simulink library "ADCS_lib"  (R2019a)
settings: Solver=VariableStepAuto  StartTime=0.0  StopTime=10.0  RelTol=1e-3
undefined symbols (not defined in the file): D_distri, G_g, G_s, G_t, Gs, I_rw, I_vscmg, I_w, J_w, K, Kc, Ki, Kp, Kv, m, OMEGA_0, P, quat_0, smiData, X, Y, Z
libraries: sm_lib x31, aerolibutil x15, nesl_utility x13, sharedtransform x4, $bdroot x2
(part 3 of 3)

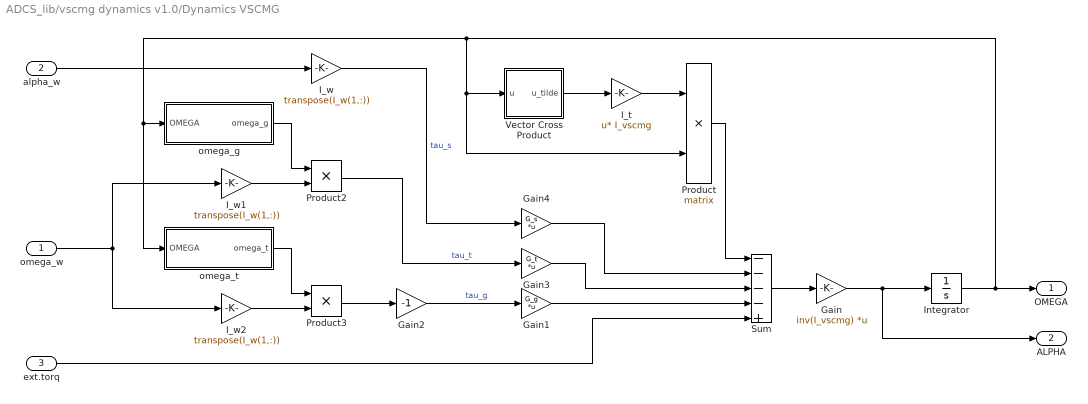
== system ADCS_lib/vscmg dynamics v1.0/Dynamics VSCMG ==
  omega_w : Inport
  alpha_w : Inport  Port=2
  ext.torq : Inport  Port=3
  Gain : Gain  Gain=inv(I_vscmg)  Multiplication=Matrix(K*u)
  Gain1 : Gain  Gain=G_g  Multiplication=Matrix(K*u)
  Gain2 : Gain  Gain=-1
  Gain3 : Gain  Gain=G_t  Multiplication=Matrix(K*u)
  Gain4 : Gain  Gain=G_s  Multiplication=Matrix(K*u)
  I_t : Gain  Gain=I_vscmg  Multiplication=Matrix(u*K)
  I_w : Gain  Gain=transpose(I_w(1,:))
  I_w1 : Gain  Gain=transpose(I_w(1,:))
  I_w2 : Gain  Gain=transpose(I_w(1,:))
  Integrator : Integrator  InitialCondition=OMEGA_0
  Product : Product  Multiplication=Matrix(*)
  Product2 : Product
  Product3 : Product
  Sum : Sum  Inputs=----+
  Vector Cross Product : MATLAB Function  TreatAsAtomicUnit=on
  omega_g : Subsystem
  omega_t : Subsystem
  OMEGA : Outport
  ALPHA : Outport  Port=2
  wires:
  Sum/1 -> Gain/1
  Gain/1 -> Integrator/1, ALPHA/1
  Integrator/1 -> omega_g/1(OMEGA), omega_t/1(OMEGA), Product/2, Vector Cross Product/1(u), OMEGA/1
  Vector Cross Product/1(u_tilde) -> I_t/1
  I_t/1 -> Product/1
  Product/1 -> Sum/1
  ext.torq/1 -> Sum/5
  alpha_w/1 -> I_w/1
  I_w/1 -> Gain4/1  "tau_s"
  I_w1/1 -> Product2/2
  omega_g/1(omega_g) -> Product2/1
  omega_t/1(omega_t) -> Product3/1
  I_w2/1 -> Product3/2
  omega_w/1 -> I_w1/1, I_w2/1
  Product3/1 -> Gain2/1
  Gain2/1 -> Gain1/1  "tau_g"
  Product2/1 -> Gain3/1  "tau_t"
  Gain1/1 -> Sum/4
  Gain3/1 -> Sum/3
  Gain4/1 -> Sum/2

== system ADCS_lib/vscmg dynamics v1.0/Kinematics1 ==
  OMEGA : Inport
  Constant : Constant  Value=0
  Gain : Gain  Gain=0.5
  Integrator : Integrator  InitialCondition=quat_0
  Quaternion Multiplication : aerolibutil/Quaternion Multiplication
  Vector Concatenate : Concatenate
  q : Outport
  wires:
  Constant/1 -> Vector Concatenate/1
  Vector Concatenate/1 -> Quaternion Multiplication/2
  Gain/1 -> Quaternion Multiplication/1
  Integrator/1 -> Gain/1, q/1
  OMEGA/1 -> Vector Concatenate/2
  Quaternion Multiplication/1 -> Integrator/1

== system ADCS_lib/vscmg dynamics v1.0/VSCMGC ==
  ALPHA : Inport
  tau_cmd : Inport  Port=2
  Demux : Demux
  Distri Mtx2 : Gain  Gain=D_distri  Multiplication=Matrix(K*u)
  Mux1 : Mux
  Mux2 : Mux
  RW 1 : Subsystem
  RW 2 : Subsystem
  RW 3 : Subsystem
  RW 4 : Subsystem
  omega_w : Outport
  alpha_w : Outport  Port=2
  wires:
  Demux/3 -> RW 3/2(u_s_3)
  Demux/1 -> RW 1/2(u_s_1)
  Demux/2 -> RW 2/2(u_s_2)
  Demux/4 -> RW 4/2(u_s_4)
  tau_cmd/1 -> Distri Mtx2/1
  ALPHA/1 -> RW 4/1(ALPHA), RW 3/1(ALPHA), RW 2/1(ALPHA), RW 1/1(ALPHA)
  Distri Mtx2/1 -> Demux/1  "u_s"
  Mux1/1 -> alpha_w/1
  Mux2/1 -> omega_w/1
  RW 1/1(omega_w_1) -> Mux2/1
  RW 2/1(omega_w_2) -> Mux2/2
  RW 3/1(omega_w_3) -> Mux2/3
  RW 4/1(omega_w_4) -> Mux2/4
  RW 1/2(alpha_w_1) -> Mux1/1
  RW 2/2(alpha_w_2) -> Mux1/2
  RW 3/2(alpha_w_3) -> Mux1/3
  RW 4/2(alpha_w_4) -> Mux1/4

== system ADCS_lib/Actuator/Reaction Wheel Cluster/RW 1 ==
  OMEGA : Inport
  ALPHA : Inport  Port=2
  u_s_1 : Inport  Port=3
  Gain : Gain  Gain=1/I_w(1,1)
  Gain1 : Gain  Gain=G_s(:,1).'  Multiplication=Matrix(K*u)
  Gain2 : Gain  Gain=G_s(:,1).'  Multiplication=Matrix(K*u)
  I_w : Gain  Gain=I_w(1,1)
  Integrator : Integrator
  Sum : Sum  Inputs=+-
  Sum1 : Sum
  h_w_1 : Outport
  omega_w_1 : Outport  Port=2
  wires:
  Sum/1 -> Integrator/1
  Integrator/1 -> Sum1/2, omega_w_1/1
  u_s_1/1 -> Gain/1
  Gain/1 -> Sum/1
  Gain1/1 -> Sum/2
  ALPHA/1 -> Gain1/1
  Sum1/1 -> I_w/1
  I_w/1 -> h_w_1/1
  Gain2/1 -> Sum1/1
  OMEGA/1 -> Gain2/1

== system ADCS_lib/Actuator/Reaction Wheel Cluster/RW 2 ==
  OMEGA : Inport
  ALPHA : Inport  Port=2
  u_s_2 : Inport  Port=3
  Gain : Gain  Gain=1/I_w(1,2)
  Gain1 : Gain  Gain=G_s(:,2).'  Multiplication=Matrix(K*u)
  Gain2 : Gain  Gain=G_s(:,2).'  Multiplication=Matrix(K*u)
  I_w : Gain  Gain=I_w(1,2)
  Integrator : Integrator
  Sum : Sum  Inputs=+-
  Sum1 : Sum
  h_w_2 : Outport
  omega_w_2 : Outport  Port=2
  wires:
  OMEGA/1 -> Gain2/1
  Gain2/1 -> Sum1/1
  I_w/1 -> h_w_2/1
  Sum1/1 -> I_w/1
  ALPHA/1 -> Gain1/1
  Gain1/1 -> Sum/2
  Gain/1 -> Sum/1
  u_s_2/1 -> Gain/1
  Integrator/1 -> omega_w_2/1, Sum1/2
  Sum/1 -> Integrator/1

== system ADCS_lib/Actuator/Reaction Wheel Cluster/RW 3 ==
  OMEGA : Inport
  ALPHA : Inport  Port=2
  u_s_3 : Inport  Port=3
  Gain : Gain  Gain=1/I_w(1,3)
  Gain1 : Gain  Gain=G_s(:,3).'  Multiplication=Matrix(K*u)
  Gain2 : Gain  Gain=G_s(:,3).'  Multiplication=Matrix(K*u)
  I_w : Gain  Gain=I_w(1,3)
  Integrator : Integrator
  Sum : Sum  Inputs=+-
  Sum1 : Sum
  h_w_3 : Outport
  omega_w_3 : Outport  Port=2
  wires:
  Sum/1 -> Integrator/1
  Integrator/1 -> Sum1/2, omega_w_3/1
  u_s_3/1 -> Gain/1
  Gain/1 -> Sum/1
  Gain1/1 -> Sum/2
  ALPHA/1 -> Gain1/1
  Sum1/1 -> I_w/1
  I_w/1 -> h_w_3/1
  Gain2/1 -> Sum1/1
  OMEGA/1 -> Gain2/1

== system ADCS_lib/Actuator/Reaction Wheel Cluster/RW 4 ==
  OMEGA : Inport
  ALPHA : Inport  Port=2
  u_s_4 : Inport  Port=3
  Gain : Gain  Gain=1/I_w(1,4)
  Gain1 : Gain  Gain=G_s(:,4).'  Multiplication=Matrix(K*u)
  Gain2 : Gain  Gain=G_s(:,4).'  Multiplication=Matrix(K*u)
  I_w : Gain  Gain=I_w(1,4)
  Integrator : Integrator
  Sum : Sum  Inputs=+-
  Sum1 : Sum
  h_w_4 : Outport
  omega_w_4 : Outport  Port=2
  wires:
  OMEGA/1 -> Gain2/1
  Gain2/1 -> Sum1/1
  I_w/1 -> h_w_4/1
  Sum1/1 -> I_w/1
  ALPHA/1 -> Gain1/1
  Gain1/1 -> Sum/2
  Gain/1 -> Sum/1
  u_s_4/1 -> Gain/1
  Integrator/1 -> omega_w_4/1, Sum1/2
  Sum/1 -> Integrator/1

== system ADCS_lib/LQI_Full State_Verified1/Vector Out Unwinding1/Short Rotation ==
  q : Inport
  Gain1 : Gain  Gain=-1
  Sign1 : Signum
  extract scalar part : Selector  InputPortWidth=4  IndexOptions=Index vector (dialog)  Indices=[1]  OutputSizes=1
  sgn : Outport
  wires:
  Gain1/1 -> sgn/1
  Sign1/1 -> Gain1/1
  extract scalar part/1 -> Sign1/1
  q/1 -> extract scalar part/1

== system ADCS_lib/LQI_Half State_Don't Use!/Vector Out Unwinding2/Short Rotation ==
  q : Inport
  Gain1 : Gain  Gain=-1
  Sign1 : Signum
  extract scalar part : Selector  InputPortWidth=4  IndexOptions=Index vector (dialog)  Indices=[1]  OutputSizes=1
  sgn : Outport
  wires:
  q/1 -> extract scalar part/1
  extract scalar part/1 -> Sign1/1
  Sign1/1 -> Gain1/1
  Gain1/1 -> sgn/1

== system ADCS_lib/LQR Compensated_Verified/Vector Out Unwinding/Short Rotation ==
  q : Inport
  Gain1 : Gain  Gain=-1
  Sign1 : Signum
  extract scalar part : Selector  InputPortWidth=4  IndexOptions=Index vector (dialog)  Indices=[1]  OutputSizes=1
  sgn : Outport
  wires:
  q/1 -> extract scalar part/1
  extract scalar part/1 -> Sign1/1
  Sign1/1 -> Gain1/1
  Gain1/1 -> sgn/1

== system ADCS_lib/PIV Compact_Verified/Vector Out Unwinding/Short Rotation ==
  q : Inport
  Gain1 : Gain  Gain=-1
  Sign1 : Signum
  extract scalar part : Selector  InputPortWidth=4  IndexOptions=Index vector (dialog)  Indices=[1]  OutputSizes=1
  sgn : Outport
  wires:
  q/1 -> extract scalar part/1
  extract scalar part/1 -> Sign1/1
  Sign1/1 -> Gain1/1
  Gain1/1 -> sgn/1

== system ADCS_lib/PIV Compact_Verified/Vector Out Unwinding1/Short Rotation ==
  q : Inport
  Gain1 : Gain  Gain=-1
  Sign1 : Signum
  extract scalar part : Selector  InputPortWidth=4  IndexOptions=Index vector (dialog)  Indices=[1]  OutputSizes=1
  sgn : Outport
  wires:
  Gain1/1 -> sgn/1
  Sign1/1 -> Gain1/1
  extract scalar part/1 -> Sign1/1
  q/1 -> extract scalar part/1

== system ADCS_lib/vscmg dynamics v1.0/Dynamics VSCMG/omega_g ==
  OMEGA : Inport
  Gain : Gain  Gain=transpose(G_g(:,1))  Multiplication=Matrix(K*u)
  Gain1 : Gain  Gain=transpose(G_g(:,2))  Multiplication=Matrix(K*u)
  Gain2 : Gain  Gain=transpose(G_g(:,3))  Multiplication=Matrix(K*u)
  Gain3 : Gain  Gain=transpose(G_g(:,4))  Multiplication=Matrix(K*u)
  Mux : Mux
  omega_g : Outport
  wires:
  Mux/1 -> omega_g/1
  Gain3/1 -> Mux/4
  Gain2/1 -> Mux/3
  Gain1/1 -> Mux/2
  Gain/1 -> Mux/1
  OMEGA/1 -> Gain/1, Gain1/1, Gain2/1, Gain3/1

== system ADCS_lib/vscmg dynamics v1.0/Dynamics VSCMG/omega_t ==
  OMEGA : Inport
  Gain : Gain  Gain=transpose(G_t(:,1))  Multiplication=Matrix(K*u)
  Gain1 : Gain  Gain=transpose(G_t(:,2))  Multiplication=Matrix(K*u)
  Gain2 : Gain  Gain=transpose(G_t(:,3))  Multiplication=Matrix(K*u)
  Gain3 : Gain  Gain=transpose(G_t(:,4))  Multiplication=Matrix(K*u)
  Mux : Mux
  omega_t : Outport
  wires:
  OMEGA/1 -> Gain3/1, Gain2/1, Gain1/1, Gain/1
  Gain/1 -> Mux/1
  Gain1/1 -> Mux/2
  Gain2/1 -> Mux/3
  Gain3/1 -> Mux/4
  Mux/1 -> omega_t/1

== system ADCS_lib/vscmg dynamics v1.0/VSCMGC/RW 1 ==
  ALPHA : Inport
  u_s_1 : Inport  Port=2
  Gain : Gain  Gain=1/I_w(1,1)
  Gain1 : Gain  Gain=G_s(:,1).'  Multiplication=Matrix(K*u)
  Integrator : Integrator
  Sum : Sum  Inputs=+-
  omega_w_1 : Outport
  alpha_w_1 : Outport  Port=2
  wires:
  Sum/1 -> alpha_w_1/1, Integrator/1
  Integrator/1 -> omega_w_1/1
  u_s_1/1 -> Gain/1
  Gain/1 -> Sum/1
  Gain1/1 -> Sum/2
  ALPHA/1 -> Gain1/1

== system ADCS_lib/vscmg dynamics v1.0/VSCMGC/RW 2 ==
  ALPHA : Inport
  u_s_2 : Inport  Port=2
  Gain : Gain  Gain=1/I_w(1,2)
  Gain1 : Gain  Gain=G_s(:,2).'  Multiplication=Matrix(K*u)
  Integrator : Integrator
  Sum : Sum  Inputs=+-
  omega_w_2 : Outport
  alpha_w_2 : Outport  Port=2
  wires:
  ALPHA/1 -> Gain1/1
  Gain1/1 -> Sum/2
  Gain/1 -> Sum/1
  u_s_2/1 -> Gain/1
  Integrator/1 -> omega_w_2/1
  Sum/1 -> alpha_w_2/1, Integrator/1

== system ADCS_lib/vscmg dynamics v1.0/VSCMGC/RW 3 ==
  ALPHA : Inport
  u_s_3 : Inport  Port=2
  Gain : Gain  Gain=1/I_w(1,3)
  Gain1 : Gain  Gain=G_s(:,3).'  Multiplication=Matrix(K*u)
  Integrator : Integrator
  Sum : Sum  Inputs=+-
  omega_w_3 : Outport
  alpha_w_3 : Outport  Port=2
  wires:
  Sum/1 -> alpha_w_3/1, Integrator/1
  Integrator/1 -> omega_w_3/1
  u_s_3/1 -> Gain/1
  Gain/1 -> Sum/1
  Gain1/1 -> Sum/2
  ALPHA/1 -> Gain1/1

== system ADCS_lib/vscmg dynamics v1.0/VSCMGC/RW 4 ==
  ALPHA : Inport
  u_s_4 : Inport  Port=2
  Gain : Gain  Gain=1/I_w(1,4)
  Gain1 : Gain  Gain=G_s(:,4).'  Multiplication=Matrix(K*u)
  Integrator : Integrator
  Sum : Sum  Inputs=+-
  omega_w_4 : Outport
  alpha_w_4 : Outport  Port=2
  wires:
  ALPHA/1 -> Gain1/1
  Gain1/1 -> Sum/2
  Gain/1 -> Sum/1
  u_s_4/1 -> Gain/1
  Integrator/1 -> omega_w_4/1
  Sum/1 -> alpha_w_4/1, Integrator/1

== matlab function ADCS_lib/Reaction Wheel ==
  data: ALPHA input; tau_wheel output; u_s_cmd input; index input; omega_wheel output; h_wheel output
function [tau_wheel,omega_wheel,h_wheel] = RW(ALPHA,u_s_cmd,index)

tau_wheel = u_s_cmd-J_w(1,index)*(transpose(Gs(:,index))*ALPHA);
omega_wheel = (tau_wheel^2)/(2*J_w(1,index));
h_wheel = J_w(1,index)*omega_wheel;

== matlab function ADCS_lib/QuEST ==
  data: V_N input; BN output size=[4 1]; V_B input; WT input
function BN = quest(V_N,V_B,WT)
B = zeros(3);

% count # of sensors
dim = size(V_N); 
n_sensor = dim(2);

% normalize V_N
for n = 1:n_sensor
    V_N(:,n)=V_N(:,n)/norm(V_N(:,n));
end
    
% normalize V_B
for n = 1:n_sensor
    V_B(:,n)=V_B(:,n)/norm(V_B(:,n));
end

% assemble K matrix
for n = 1:n_sensor
    B=WT(n)*V_B(:,n)*transpose(V_N(:,n))+B;
end
S = B+transpose(B);
sigma = trace(B);
Z = [B(2,3)-B(3,2);
     B(3,1)-B(1,3);
     B(1,2)-B(2,1)];
K = [sigma transpose(Z);Z S-sigma*eye(3)];

% optimize eigenvalue
lambda = sum(WT); % first guess
for i = 1:2
    f = det(K-lambda*eye(4));
    f_dash = det(K-lambda*eye(4))*trace(inv(K-lambda*eye(4))*-eye(4));
    lambda = lambda - (f/f_dash);
end

% compute Rodrigues parameter & convert to Quaternion
q = inv((lambda+sigma)*eye(3)-S)*Z;
quatr = [1;q]/sqrt(1+transpose(q)*q);

BN = quatr;

== matlab function ADCS_lib/Reaction Wheel Cluster/Reaction Wheel 1 ==
  data: ALPHA input; tau_wheel output; u_s_cmd input; index input; omega_wheel output; h_wheel output
function [tau_wheel,omega_wheel,h_wheel] = RW(ALPHA,u_s_cmd,index)

tau_wheel = u_s_cmd-J_w(1,index)*(transpose(Gs(:,index))*ALPHA);
omega_wheel = (tau_wheel^2)/(2*J_w(1,index));
h_wheel = J_w(1,index)*omega_wheel;

== matlab function ADCS_lib/Reaction Wheel Cluster/Reaction Wheel 2 ==
  data: ALPHA input; tau_wheel output; u_s_cmd input; index input; omega_wheel output; h_wheel output
function [tau_wheel,omega_wheel,h_wheel] = RW(ALPHA,u_s_cmd,index)

tau_wheel = u_s_cmd-J_w(1,index)*(transpose(Gs(:,index))*ALPHA);
omega_wheel = (tau_wheel^2)/(2*J_w(1,index));
h_wheel = J_w(1,index)*omega_wheel;

== matlab function ADCS_lib/Reaction Wheel Cluster/Reaction Wheel 3 ==
  data: ALPHA input; tau_wheel output; u_s_cmd input; index input; omega_wheel output; h_wheel output
function [tau_wheel,omega_wheel,h_wheel] = RW(ALPHA,u_s_cmd,index)

tau_wheel = u_s_cmd-J_w(1,index)*(transpose(Gs(:,index))*ALPHA);
omega_wheel = (tau_wheel^2)/(2*J_w(1,index));
h_wheel = J_w(1,index)*omega_wheel;

== matlab function ADCS_lib/Reaction Wheel Cluster/Reaction Wheel 4 ==
  data: ALPHA input; tau_wheel output; u_s_cmd input; index input; omega_wheel output; h_wheel output
function [tau_wheel,omega_wheel,h_wheel] = RW(ALPHA,u_s_cmd,index)

tau_wheel = u_s_cmd-J_w(1,index)*(transpose(Gs(:,index))*ALPHA);
omega_wheel = (tau_wheel^2)/(2*J_w(1,index));
h_wheel = J_w(1,index)*omega_wheel;

== matlab function ADCS_lib/tilde_cross P ==
  data: u input; u_tilde output
function u_tilde = tilde(u)
u_tilde = [0 -u(3) u(2);
           u(3) 0 -u(1);
           -u(2) u(1) 0];

== matlab function ADCS_lib/Satellite Dynamics/Equation of Motion ==
  data: OMEGA input; ALPHA output; h_app_RWC input; tau_app_RWC input; tau_app_distrb input
function ALPHA = dynamics(OMEGA,h_app_RWC,tau_app_RWC,tau_app_distrb)

% assemble OMEGA_tilde for cross product
OMEGA_tilde = [0 -OMEGA(3) OMEGA(2);
               OMEGA(3) 0 -OMEGA(1);
              -OMEGA(2) OMEGA(1) 0];
          
% calculate ALPHA
ALPHA = inv(I_tot) * (-OMEGA_tilde*I_tot*OMEGA - tau_app_RWC - OMEGA_tilde*h_app_RWC + tau_app_distrb)

== matlab function ADCS_lib/Dynamics1/Vector Cross Product ==
  data: u input; u_tilde output
function u_tilde = tilde(u)
u_tilde = [0 -u(3) u(2);
           u(3) 0 -u(1);
           -u(2) u(1) 0];

== matlab function ADCS_lib/Dynamics/Vector Cross Product ==
  data: u input; u_tilde output
function u_tilde = tilde(u)
u_tilde = [0 -u(3) u(2);
           u(3) 0 -u(1);
           -u(2) u(1) 0];

== matlab function ADCS_lib/Dynamics/Vector Cross Product1 ==
  data: u input; u_tilde output
function u_tilde = tilde(u)
u_tilde = [0 -u(3,1) u(2,1);
           u(3,1) 0 -u(1,1);
           -u(2,1) u(1,1) 0];

== matlab function ADCS_lib/Dynamics1/Vector Cross Product1 ==
  data: u input; u_tilde output
function u_tilde = tilde(u)
u_tilde = [0 -u(3,1) u(2,1);
           u(3,1) 0 -u(1,1);
           -u(2,1) u(1,1) 0];

== matlab function ADCS_lib/FeedFwd/Vector Cross Product ==
  data: u input; u_tilde output
function u_tilde = tilde(u)
u_tilde = [0 -u(3) u(2);
           u(3) 0 -u(1);
           -u(2) u(1) 0];

== matlab function ADCS_lib/vscmg dynamics v1.0/Dynamics VSCMG/Vector Cross Product ==
  data: u input; u_tilde output
function u_tilde = tilde(u)
u_tilde = [0 -u(3) u(2);
           u(3) 0 -u(1);
           -u(2) u(1) 0];

== matlab function ADCS_lib/FeedFwd/Vector Cross Product1 ==
  data: u input; u_tilde output
function u_tilde = tilde(u)
u_tilde = [0 -u(3,1) u(2,1);
           u(3,1) 0 -u(1,1);
           -u(2,1) u(1,1) 0];

== matlab function ADCS_lib/PV Full EoM Ctrl/Vector Cross Product ==
  data: u input; u_tilde output
function u_tilde = tilde(u)
u_tilde = [0 -u(3) u(2);
           u(3) 0 -u(1);
           -u(2) u(1) 0];
